simulink library "unitConverter_Lib"  (Simulink 7.8)
settings: Solver=ode45  StartTime=0.0  StopTime=10.0  RelTol=1e-3
settings Model: Creator=vpadmaj  LastModifiedBy=VPADMAJ

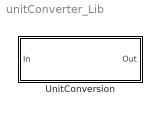
== system unitConverter_Lib ==
  UnitConversion : Subsystem  mask(UnitConversion){Selection=°C_to_K, Gain_User=0, Offset_User=[]}
      mask prompts: Selection "ConversionReqd"; Gain_User "Gain"; Offset_User "Offset"
      mask help:
      | Conversions available:
      | °C_to_K
      | degC_to_degK
      | K_to_°C
      | degK_to_degC
      | hPa_to_bar
      | bar_to_hPa
      | g/min_to_kg/s
      | kg/s_to_g/min
      | kg/h_to_kg/s
      | kg/s_to_kg/h
      | km/h_to_m/s
      | m/s_to_km/h
      | rpm_to_%
      | %_to_rpm
      | deg_to_steps
      | steps_to_deg
      | steps_to_bit
      | bit_to_steps
      |
      | Please remove this block and insert appropriate maps for 'rpm_to_%' and
      | 'deg_to_steps'
      mask init:
      | switch Selection
      |     case '°C_to_K'
      |       Offset = 273.15; Gain = 1; Unit1 = '°C'; Unit2 = 'K';
      |     case 'degC_to_degK'
      |       Offset = 273.15; Gain = 1; Unit1 = '°C'; Unit2 = 'K';
      |     case 'K_to_°C'
      |       Offset = -273.15; Gain = 1; Unit1 = 'K'; Unit2 = '°C';
      |     case 'degK_to_degC'
      |       Offset = -273.15; Gain = 1; Unit1 = 'K'; Unit2 = '°C';
      |     case 'hPa_to_bar'
      |       Offset = 0; Gain = 1/1000; Unit1 = 'hPa'; Unit2 = 'bar';
      |     case 'bar_to_hPa'
      |       Offset = 0; Gain = 1000; Unit1 = 'bar'; Unit2 = 'hPa';
      |     case 'g/min_to_kg/s'
      |       Offset = 0; Gain = 1/60000; Unit1 = 'g/min'; Unit2 = 'kg/s';
      |     case 'kg/s_to_g/min'
      |       Offset = 0; Gain = 60000; Unit1 = 'kg/s'; Unit2 = 'g/min';
      |     case 'kg/h_to_kg/s'
      |       Offset = 0; Gain = 1/3600; Unit1 = 'kg/h'; Unit2 = 'kg/s';
      |     case 'kg/s_to_kg/h'
      |        Offset = 0; Gain = 3600; Unit1 = 'kg/s'; Unit2 = 'kg/h';
      |     case 'km/h_to_m/s'
      |       Offset = 0; Gain = 1/3.6; Unit1 = 'km/h'; Unit2 = 'm/s';
      |     case 'm/s_to_km/h'
      |       Offset = 0; Gain = 3.6; Unit1 = 'm/s'; Unit2 = 'km/h';
      |     case 'rpm_to_%'
      |         Offset = 0; Gain = 1; Unit1 = 'rpm'; Unit2 = '%';
      |     case '%_to_rpm'
      |          Offset = 0; Gain = 1; Unit1 = '%'; Unit2 = 'rpm';
      |     case 'deg_to_steps'
      |         Offset = 0; Gain = 1; Unit1 = 'deg'; Unit2 = 'steps';
      |     case 'steps_to_deg'
      |          Offset = 0; Gain = 1; Unit1 = 'steps'; Unit2 = 'deg';
      |     case 'steps_to_bit'
      |         Offset = 0; Gain = 1; Unit1 = 'steps'; Unit2 = 'bit';
      |     case 'bit_to_steps'
      |         Offset = 0; Gain = 1; Unit1 = 'bit'; Unit2 = 'steps';
      |     case 'Others'
      |       Offset = Offset_User; Gain = Gain_User; Unit1 = '-'; Unit2 = '-';
      |     case 'NoConversionReqd'
      |       Offset = 0; Gain = 1; Unit1 = ' '; Unit2 = ' ';
      |     otherwise
      |       Offset = 0; Gain = 1; Unit1 = ' '; Unit2 = ' ';
      | end
      mask StyleString: popup(°C_to_K|degC_to_degK|K_to_°C|degK_to_degC|hPa_to_bar|bar_to_hPa|g/min_to_kg/s|kg/s_to_g/min|kg/h_to_kg/s|kg/s_to_kg/h|km/h_to_m/s|m/s_to_km/h|rpm_to_%|%_to_rpm|deg_to_steps|steps_to_deg|steps_to_bit|bit_to_steps|Others|NoConversionReqd),edit,edit
      mask Display:
      | % port_label('input',1,['[', Unit1, ']- [ Gain:', Gain])
      | % port_label('output',1, [' ; Offset: ', Offset,'] [', Unit2, ']'])
      | fprintf('%s_to_%s \n [Gain:%s]  \n [Offset:%s]',Unit1, Unit2, num2str(Gain), num2str(Offset))

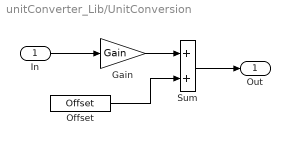
== system unitConverter_Lib/UnitConversion ==
  In : Inport  Tag=inport
  Gain : Gain  Tag=u2_  Gain=Gain  SaturateOnIntegerOverflow=on  OutDataTypeStr=Inherit: Same as input  ParamDataTypeStr=Inherit: Same as input
  Offset : Constant  Tag=offset_  Value=Offset
  Sum : Sum  SaturateOnIntegerOverflow=on  InputSameDT=on  OutDataTypeStr=Inherit: Same as first input
  Out : Outport  Tag=outport
  wires:
  Sum/1 -> Out/1
  Gain/1 -> Sum/1
  Offset/1 -> Sum/2
  In/1 -> Gain/1
